simulink subsystem "Subsystem1"  (R2019b)
settings: Solver=VariableStepAuto  StartTime=0.0  StopTime=10.0  RelTol=1e-3
values from neighbouring files (symbols this model uses):
  x0 = [0, 0, 0.05, 2, 0, 0.01, 0.02, 0, 0, 0, 0, 0]    [createmodels.m]    (also in pidcontrolstartupscript.m = [0, 0, 0.05, 8, 0, 0.01, 0.02, 0, 0, 0, 0, 0])
undefined symbols (not defined in the file or in its folder): scalemodelstatefunction
libraries: aerolibanim x1
settings Model: Creator=Vlad  LastModifiedBy=Vlad

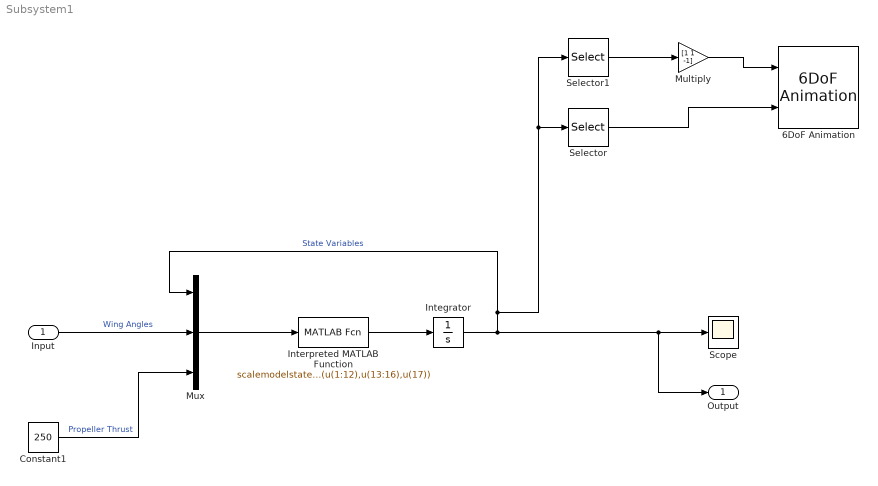
== system Subsystem1 ==
  Input : Inport
  6DoF Animation : aerolibanim/6DoF Animation  u1=[0 30 -2 2 0 1]  u2=0.1  u3=5  u4=[4000 0 -5000]  u5=Fixed position  u6=[20 20 20]  u7=10  u8=on
      settings: SourceProductName=Aerospace Blockset
  Constant1 : Constant  Value=250
  Integrator : Integrator  InitialCondition=x0
  Interpreted MATLAB Function : MATLABFcn  MATLABFcn=scalemodelstatefunction(u(1:12),u(13:16),u(17))  OutputDimensions=12
  Multiply : Gain  Gain=[1 1 -1]
  Mux : Mux  Inputs=3
  Scope : Scope
  Selector : Selector  InputPortWidth=12  IndexOptions=Index vector (dialog)  Indices=[8 7 9]  OutputSizes=1
  Selector1 : Selector  InputPortWidth=12  IndexOptions=Index vector (dialog)  Indices=[1 2 3]  OutputSizes=1
  Output : Outport
  wires:
  Mux/1 -> Interpreted MATLAB Function/1
  Input/1 -> Mux/2  "Wing Angles"
  Constant1/1 -> Mux/3  "Propeller Thrust"
  Multiply/1 -> 6DoF Animation/1
  Interpreted MATLAB Function/1 -> Integrator/1
  Integrator/1 -> Mux/1, Selector/1, Selector1/1, Scope/1, Output/1  "State Variables"
  Selector/1 -> 6DoF Animation/2
  Selector1/1 -> Multiply/1
